simulink model "A1_sim"  (R2020b)
settings: Solver=ode5  StartTime=0.0  StopTime=200  FixedStep=0.001  RelTol=1e-3
values from neighbouring files (symbols this model uses):
  J = diag([700,700,500])    [A1.m]
undefined symbols (not defined in the file or in its folder): K
libraries: vrlib x2
settings Model: Creator=mirrormire  LastModifiedBy=mirrormire

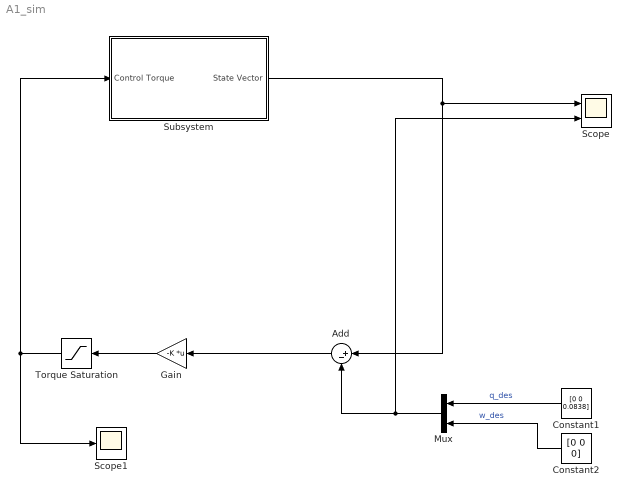
== system A1_sim ==
  Add : Sum  Inputs=|+-
  Constant1 : Constant  Value=[0 0 0.0838]
  Constant2 : Constant  Value=[0 0 0]
  Gain : Gain  Gain=-K  Multiplication=Matrix(K*u)
  Mux : Mux  Inputs=2
  Scope : Scope  NumInputPorts=2
  Scope1 : Scope
  Subsystem : Subsystem
  Torque Saturation : Saturate  UpperLimit=2  LowerLimit=-2
  wires:
  Gain/1 -> Torque Saturation/1
  Mux/1 -> Scope/2, Add/2
  Constant1/1 -> Mux/1  "q_des"
  Constant2/1 -> Mux/2  "w_des"
  Torque Saturation/1 -> Scope1/1, Subsystem/1(Control Torque)
  Add/1 -> Gain/1
  Subsystem/1(State Vector) -> Add/1, Scope/1

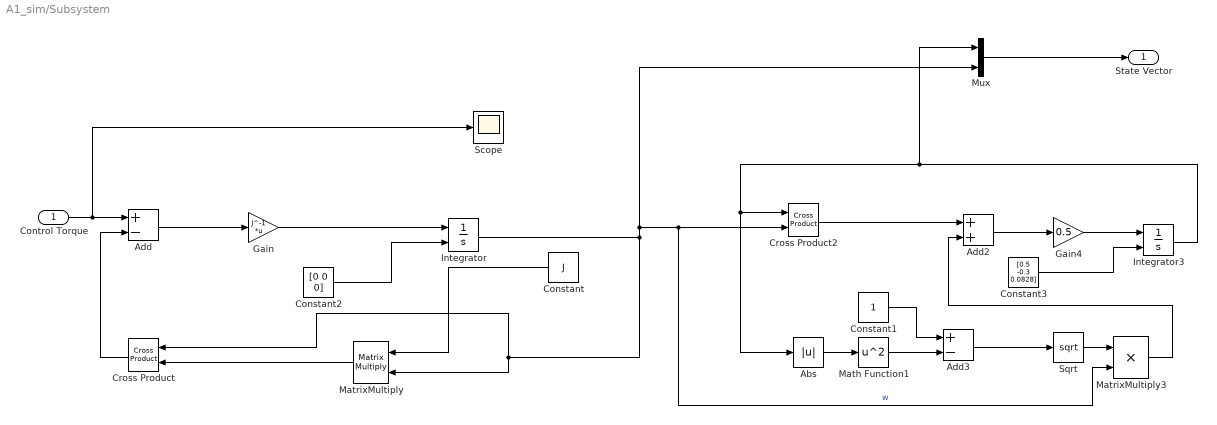
== system A1_sim/Subsystem ==
  Control Torque : Inport
  Abs : Abs
  Add : Sum  Inputs=+-
  Add2 : Sum
  Add3 : Sum  Inputs=+-
  Constant : Constant  Value=J
  Constant1 : Constant
  Constant2 : Constant  Value=[0 0 0]
  Constant3 : Constant  Value=[0.5 -0.3 0.0828]
  Cross Product : vrlib/Utilities/Cross Product
  Cross Product2 : vrlib/Utilities/Cross Product
  Gain : Gain  Gain=J^-1  Multiplication=Matrix(K*u)
  Gain4 : Gain  Gain=0.5
  Integrator : Integrator  InitialConditionSource=external
  Integrator3 : Integrator  InitialConditionSource=external
  Math Function1 : Math  Operator=square  SaturateOnIntegerOverflow=on
  MatrixMultiply : Product  Multiplication=Matrix(*)
  MatrixMultiply3 : Product
  Mux : Mux  Inputs=2
  Scope : Scope
  Sqrt : Sqrt  SaturateOnIntegerOverflow=on
  State Vector : Outport
  wires:
  Mux/1 -> State Vector/1
  Gain/1 -> Integrator/1
  Constant/1 -> MatrixMultiply/1
  Cross Product/1 -> Add/2
  Control Torque/1 -> Scope/1, Add/1
  Add/1 -> Gain/1
  MatrixMultiply/1 -> Cross Product/2
  Integrator/1 -> MatrixMultiply3/2, Cross Product2/2, Mux/2, Cross Product/1, MatrixMultiply/2  "w"
  Constant1/1 -> Add3/1
  Add2/1 -> Gain4/1
  Gain4/1 -> Integrator3/1
  Math Function1/1 -> Add3/2
  Sqrt/1 -> MatrixMultiply3/1
  Integrator3/1 -> Mux/1, Abs/1, Cross Product2/1
  MatrixMultiply3/1 -> Add2/2
  Abs/1 -> Math Function1/1
  Cross Product2/1 -> Add2/1
  Add3/1 -> Sqrt/1
  Constant2/1 -> Integrator/2
  Constant3/1 -> Integrator3/2
